simulink model "ukol_2_model"  (R2016a)
settings: Solver=VariableStepAuto  SolverMode=SingleTasking  StartTime=0.0  StopTime=100  MaxStep=1e-2  RelTol=1e-3
undefined symbols (not defined in the file): K
libraries: cstblocks x1
settings Model: Creator=tomas  LastModifiedBy=tomas
settings DebuggingCC: SFUnexpectedBacktrackingDiag=error  SFNoUnconditionalDefaultTransitionDiag=error
settings GRTTargetCC: TargetLangStandard=C99 (ISO)  GeneratePreprocessorConditionals=Use local settings
settings ConfigComp: CovMetricSettings=dwe  CovHtmlReporting=off  CovSaveCumulativeToWorkspaceVar=off  CovSaveSingleToWorkspaceVar=off  CovExternalEMLEnable=on

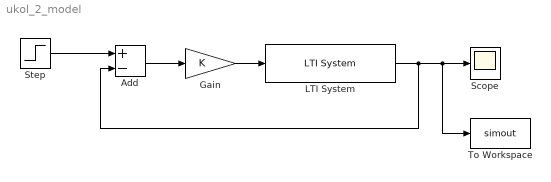
== system ukol_2_model ==
  Add : Sum  Inputs=+-
  Gain : Gain  Gain=K
  LTI System : cstblocks/LTI System  sys=Fs_servo  IC=[]
  Scope : Scope
  Step : Step  SampleTime=0
  To Workspace : ToWorkspace  VariableName=simout  SaveFormat=Timeseries  SampleTime=-1
  wires:
  Gain/1 -> LTI System/1
  LTI System/1 -> Add/2, To Workspace/1, Scope/1
  Add/1 -> Gain/1
  Step/1 -> Add/1
